simulink model "cpg_funciones"  (R2023b)
settings: Solver=ode4  StartTime=0.0  StopTime=inf  FixedStep=0.01  RelTol=1e-3
undefined symbols (not defined in the file or in its folder): CI
settings Model: Creator=KAREN  LastModifiedBy=rodri

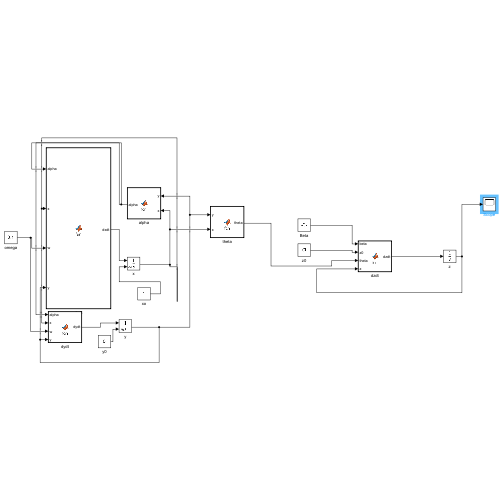
[thumbnail: Simulink's stored preview of the top-level diagram]
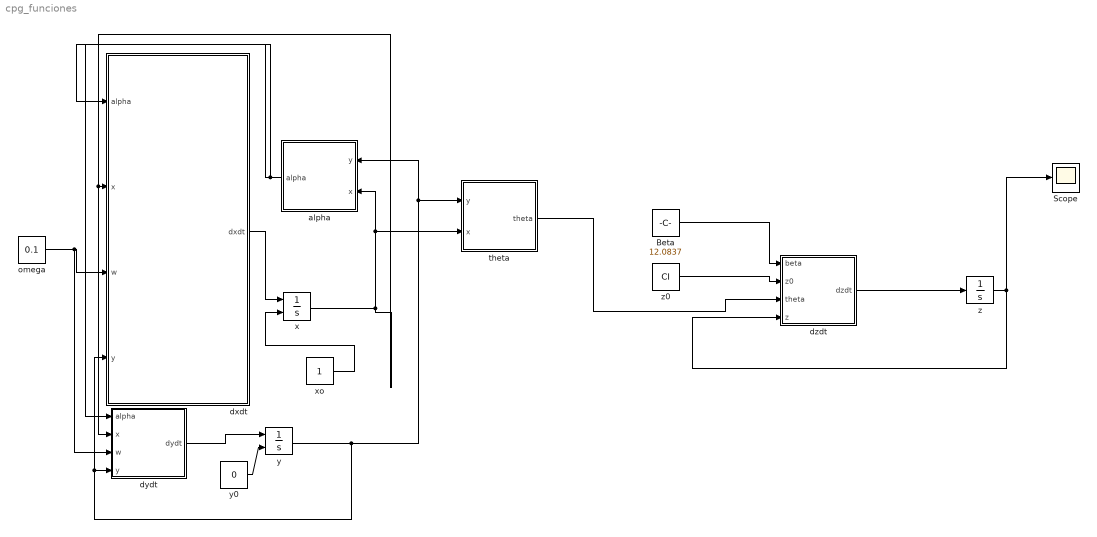
== system cpg_funciones ==
  Beta : Constant  Value=12.0837
  Scope : Scope
  alpha : MATLAB Function  TreatAsAtomicUnit=on
  dxdt : MATLAB Function  TreatAsAtomicUnit=on
  dydt : MATLAB Function  TreatAsAtomicUnit=on
  dzdt : MATLAB Function  TreatAsAtomicUnit=on
  "omega " : Constant  Value=0.1
  "theta " : MATLAB Function  TreatAsAtomicUnit=on
  x : Integrator  InitialConditionSource=external  InitialCondition=1
  "xo " : Constant
  y : Integrator  InitialConditionSource=external  InitialCondition=1
  "y0 " : Constant  Value=0
  z : Integrator
  z0 : Constant  Value=CI
  wires:
  alpha/1(alpha) -> dydt/1(alpha), dxdt/1(alpha)
  Beta/1 -> dzdt/1(beta)
  z/1 -> dzdt/4(z), Scope/1
  dxdt/1(dxdt) -> x/1
  dydt/1(dydt) -> y/1
  x/1 -> dydt/2(x), dxdt/2(x), "theta "/2(x), alpha/2(x)
  "y0 "/1 -> y/2
  dzdt/1(dzdt) -> z/1
  "omega "/1 -> dydt/3(w), dxdt/3(w)
  y/1 -> dydt/4(y), dxdt/4(y), "theta "/1(y), alpha/1(y)
  "theta "/1(theta) -> dzdt/3(theta)
  "xo "/1 -> x/2
  z0/1 -> dzdt/2(z0)

== matlab function cpg_funciones/dydt ==
  data: alpha input; x input; w input; y input; dydt output
function dydt = fcn(alpha, x, w, y)
dydt = alpha*y + w*x;

== matlab function cpg_funciones/dxdt ==
  data: alpha input; x input; w input; y input; dxdt output
function dxdt = fcn(alpha, x, w, y)
dxdt = alpha*x - w*y;

== matlab function cpg_funciones/dzdt ==
  data: beta input; z0 input; theta input; z input; dzdt output
function dzdt = fcn(beta,z0, theta, z)
a = [2.2897 12.4562 16.3255];
b = [9.3154 8.4272 6.1772];
thetaT = [6.1224 0.7493 0.4];
atractores = 0;
primerTermino = beta*(z - z0);
for i = 1:length(a)
    atractores =  atractores + a(i)*exp(-b(i)*abs(theta - thetaT(i)));
end
dzdt = - primerTermino + atractores;

== matlab function cpg_funciones/alpha ==
  data: y input; alpha output; x input
function alpha = fcn(y, x)

alpha = 1 - sqrt(x^2 + y ^2)

== matlab function cpg_funciones/theta  ==
  data: y input; theta output; x input
function theta = fcn(y, x)
angulo  = atan2(y, x);
if angulo <0 
    angulo = angulo + 2*pi
end
theta = angulo;
